simulink model "buckBoost_MPPT"  (R2024a)
settings: Solver=FixedStepDiscrete  StartTime=0.0  StopTime=.5  RelTol=1e-3
libraries: spsSeriesRLCBranchLib x4, spsDiodeLib x1, spsIGBTDiodeLib x1, spsPVArrayLib x1, eePwmGenerator x1, spsVoltageMeasurementLib x1, sps_lib x1
settings Model: Creator=farza  LastModifiedBy=farza

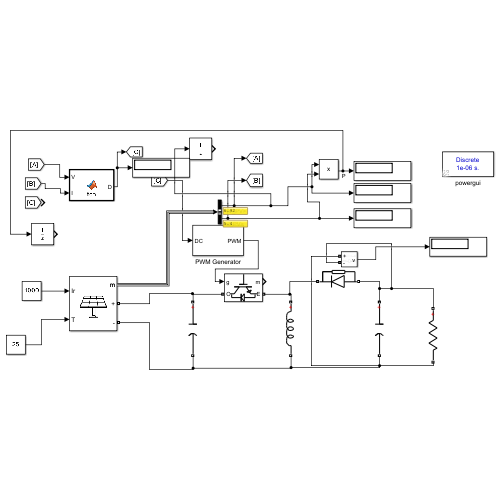
[thumbnail: Simulink's stored preview of the top-level diagram]
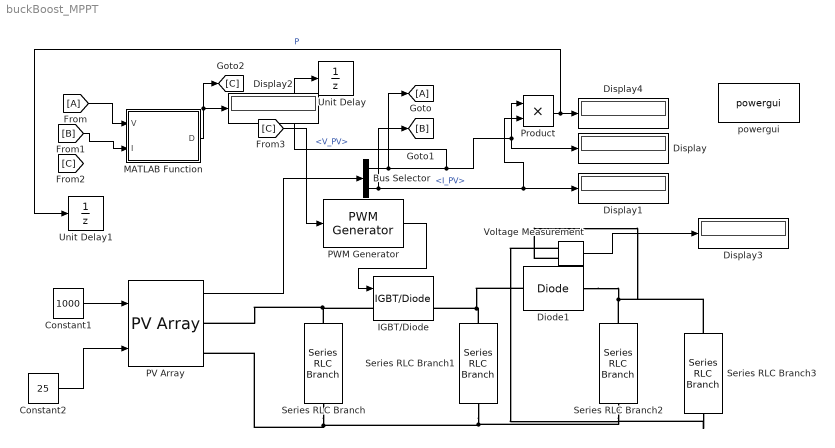
== system buckBoost_MPPT ==
  Bus Selector : BusSelector  OutputSignals=V_PV,I_PV
  Constant1 : Constant  Value=1000
  Constant2 : Constant  Value=25
  Diode1 : spsDiodeLib/Diode  Ron=0.001  Lon=0  Vf=0.8  IC=0  UseSnubber=0  Rs=500  Cs=250e-9  Measurements=off
  Display{,1..4} (5 alike) : Display
  From : From
  Goto : Goto
  IGBT/Diode : spsIGBTDiodeLib/IGBT//Diode  Ron=1e-3  Rs=1e5  Cs=inf  Measurements=on
  MATLAB Function : MATLAB Function  TreatAsAtomicUnit=on
  PV Array : spsPVArrayLib/PV Array  Npar=1  Nser=1  PlotType=array @ 1000 W/m2 & specified temperatures  S_vec="[ 1000  500  100 ]"  Temp_C_vec="[ 45 25  ]"  ModuleName=User-defined  PlotWhenSelected=off  Pm=184.7016  Ncell=72  Voc=44.14  Isc=5.43  Vm=36.72  Im=5.03  beta_Voc_pc=-0.3616  alpha_Isc_pc=0.041492  beta_Voc=-0.15961  alpha_Isc=0.002253  IL=5.4379  I0=1.8755e-10  nI=0.99182  Rsh=257.1498  Rs=0.37471  RobustModel=off  RobustCellTemperature=313.3991  BAL=on  Tc=1e-6  Tfilter=5e-5
  PWM Generator : eePwmGenerator/PWM Generator  CarrCount=Up  Tper=0.00001  Tdelay=0  Ts=1e-6
  Product : Product
  Series RLC Branch : spsSeriesRLCBranchLib/Series RLC Branch  LConnTagsString=__new0  RConnTagsString=__new0  BranchType=C  Resistance=1  Inductance=1e-3  SetiL0=off  InitialCurrent=0  Capacitance=10e-6  Setx0=off  InitialVoltage=0  Measurements=None
  Series RLC Branch1 : spsSeriesRLCBranchLib/Series RLC Branch  LConnTagsString=__new0  RConnTagsString=__new0  BranchType=L  Resistance=1  Inductance=2.233e-4  SetiL0=off  InitialCurrent=0  Capacitance=1e-6  Setx0=off  InitialVoltage=0  Measurements=None
  Series RLC Branch2 : spsSeriesRLCBranchLib/Series RLC Branch  LConnTagsString=__new0  RConnTagsString=__new0  BranchType=C  Resistance=1  Inductance=1e-3  SetiL0=off  InitialCurrent=0  Capacitance=1.445e-5  Setx0=off  InitialVoltage=0  Measurements=None
  Series RLC Branch3 : spsSeriesRLCBranchLib/Series RLC Branch  LConnTagsString=__new0  RConnTagsString=__new0  BranchType=R  Resistance=110  Inductance=1e-3  SetiL0=off  InitialCurrent=0  Capacitance=1e-6  Setx0=off  InitialVoltage=0  Measurements=None
  Unit Delay : UnitDelay  SampleTime=-1  HasFrameUpgradeWarning=on
  Unit Delay1 : UnitDelay  SampleTime=-1  HasFrameUpgradeWarning=on
  Voltage Measurement : spsVoltageMeasurementLib/Voltage Measurement  PhasorSimulation=off  OutputType=Complex  PSBequivalent=0
  powergui : sps_lib/powergui  Priority=1  SimulationMode=Discrete  SampleTime=1e-6  frequency=60  Iterations=50  frequencyindice=0  Pbase=100e6  ErrMax=1e-4  UnitsV=kV  UnitsW=MW  buscounter=0  FunctionMessages=off  echomessages=off  EnableUseOfTLC=off  CurrentSourceSwitches=off  DisableSnubberDevices=off  DisableRonSwitches=off  DisableVfSwitches=off  DisplayEquations=off  AutomaticDiscreteSolvers=off  SolverType=Tustin/Backward Euler (TBE)  Interpol=off  ExternalGateDelay=off  methode=off  Ts=100  x0status=blocks  SPID=on  SwTol=0  HookPort=off  NonlinearTolerance=1e-4  nMaxIteration=100  ContinueOnMaxIteration=off  RestoreLinks=warning  ResistiveCurrentMeasurement=off  Frange=[0:2:500]  Ylog=off  Xlog=on  ShowGrid=off  save=off  variable=ZData  structure=0  ZoomFFT=off  StartTime=0.0  cycles=1  DisplayStyle=1  fundamental=60  FreqAxis=off  MaxFrequency=1000  frequencyindicesteady=1  RmsSteady=1  display=off
  wires:
  Constant2/1 -> PV Array/2
  PV Array/1 -> Bus Selector/1
  Bus Selector/2 -> Product/2, Display1/1, [B]  "<I_PV>"
  Bus Selector/1 -> Unit Delay/1, Product/1, Display/1, Goto/1  "<V_PV>"
  Constant1/1 -> PV Array/1
  [C] -> PWM Generator/1
  Voltage Measurement/1 -> Display3/1
  PWM Generator/1 -> IGBT/Diode/1
  From/1 -> MATLAB Function/1(V)
  [B] -> MATLAB Function/2(I)
  MATLAB Function/1(D) -> [C], Display2/1
  Product/1 -> Unit Delay1/1, Display4/1  "P"
  connections:
  Series RLC Branch/LConn1 -- IGBT/Diode/LConn1 -- PV Array/RConn1
  Series RLC Branch/RConn1 -- Series RLC Branch3/RConn1 -- Voltage Measurement/LConn1 -- Series RLC Branch2/RConn1 -- Series RLC Branch1/RConn1 -- PV Array/RConn2
  Series RLC Branch1/LConn1 -- Diode1/RConn1 -- IGBT/Diode/RConn1
  Series RLC Branch2/LConn1 -- Voltage Measurement/LConn2 -- Series RLC Branch3/LConn1 -- Diode1/LConn1

== matlab function buckBoost_MPPT/MATLAB Function ==
  data: V input; D output; I input
function D = fcn(V, I)

persistent D_old P_old V_old counter
step = 0.005;
tol  = 1e-6;
N    = 50;   % print interval

if isempty(D_old)
    D_old = 0.5;
    P_old = 0;
    V_old = 0;
    counter = 0;
end

P  = V*I;
dP = P - P_old;
dV = V - V_old;

D = D_old;

if abs(dP) >= tol
    if dP > 0
        if dV > 0, D = D_old + step; else, D = D_old - step; end
    else
        if dV > 0, D = D_old - step; else, D = D_old + step; end
    end
end

% Clamp duty ratio
Dmax = 0.95;
Dmin = 0.5;
D = clamp(D,Dmin,Dmax);

% Update persistent vars
D_old = D;
P_old = P;
V_old = V;

end
